simulink model "chirp_transmit"  (R2022a)
settings: Solver=FixedStepDiscrete  StartTime=0.0  StopTime=1  FixedStep=0.10000000000000001  RelTol=1e-3
model workspace (MAT data in the model file):
  imageBits = [0 1 0 1]
settings Model: Creator=luoch  LastModifiedBy=luoch
settings DataIOCC: SaveOutput=off  SignalLogging=off
settings ModelReferenceCC: EnableRefExpFcnMdlSchedulingChecks=off
settings RTWCC: Description=Generic Real-Time Target  GPUComputeCapability=5.0
settings ConfigComp: CovBoundaryAbsTol=1.0e-5

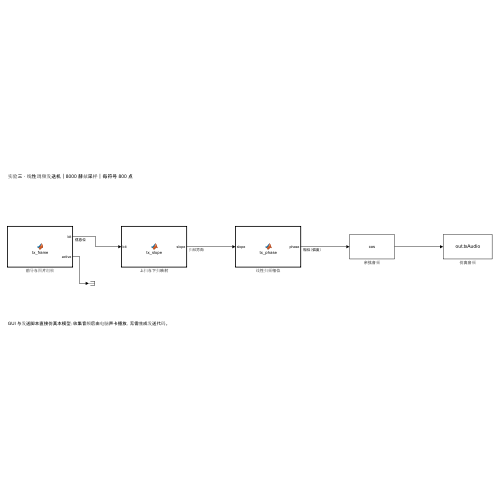
[thumbnail: Simulink's stored preview of the top-level diagram]
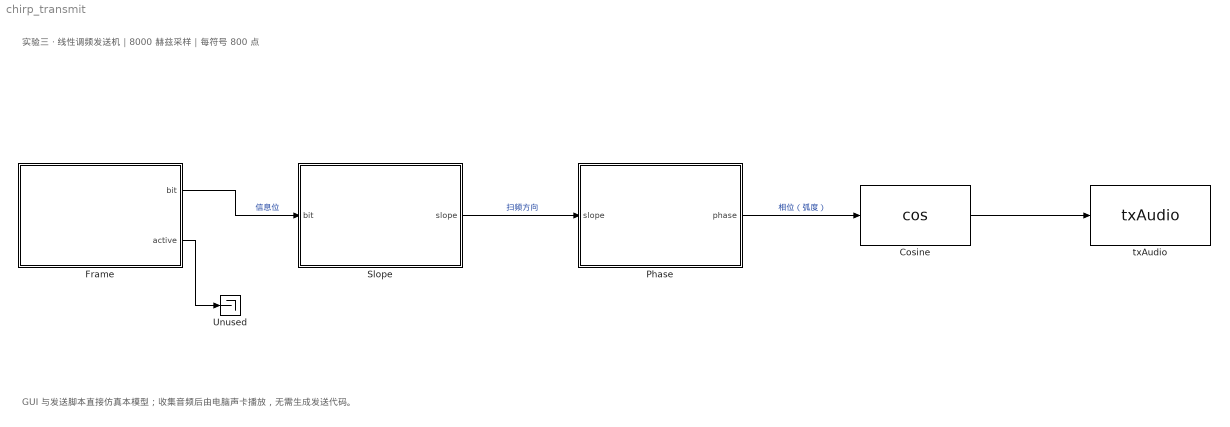
== system chirp_transmit ==
  note: 实验三 · 线性调频发送机｜8000 赫兹采样｜每符号 800 点
  note: GUI 与发送脚本直接仿真本模型；收集音频后由电脑声卡播放，无需生成发送代码。
  Cosine : Trigonometry  Operator=cos
      settings: AttributesFormatString=余弦音频
  Frame : MATLAB Function  TreatAsAtomicUnit=on
      settings: AttributesFormatString=前导与图片组帧
  Phase : MATLAB Function  TreatAsAtomicUnit=on
      settings: AttributesFormatString=线性扫频相位
  Slope : MATLAB Function  TreatAsAtomicUnit=on
      settings: AttributesFormatString=上扫与下扫映射
  Unused : Terminator
  txAudio : ToWorkspace  VariableName=txAudio  SampleTime=-1
      settings: AttributesFormatString=仿真音频
  wires:
  Frame/2(active) -> Unused/1
  Frame/1(bit) -> Slope/1(bit)  "信息位"
  Slope/1(slope) -> Phase/1(slope)  "扫频方向"
  Phase/1(phase) -> Cosine/1  "相位（弧度）"
  Cosine/1 -> txAudio/1

== matlab function chirp_transmit/Frame ==
  settings: updateMethod=DISCRETE  sampleTime=0.10000000000000001
  data: bit output; active output; imageBits parameter
function [bit,active]=tx_frame(imageBits)
%#codegen
% 前导、交替段、首尾 m 序列、图片比特及尾部保护，均在模型内产生。
persistent index
if isempty(index),index=1;end
mseq=[1 0 0 1 1 0 1 0 1 1 1 1 0 0 0];alternate=[1 0 1 0 1 0 1 0 1 0];
L=numel(imageBits);active=index<=50+L+5;bit=0;
if index>=11 && index<21,bit=alternate(index-10);
elseif index>=21 && index<36,bit=mseq(index-20);
elseif index>=36 && index<36+L,bit=imageBits(index-35);
elseif index>=36+L && index<51+L,bit=mseq(index-35-L);
end
index=index+1;
end

== matlab function chirp_transmit/Phase ==
  settings: updateMethod=DISCRETE  sampleTime=0.10000000000000001
  data: slope input; phase output
function phase=tx_phase(slope)
%#codegen
% 每符号从零相位开始；保留原实现的 800 点闭区间扫描网格。
t=linspace(0,.1,800)';phase=2*pi*1000*t+pi*slope*2000*t.^2;
end

== matlab function chirp_transmit/Slope ==
  settings: updateMethod=DISCRETE  sampleTime=0.10000000000000001
  data: bit input; slope output
function slope=tx_slope(bit)
%#codegen
% 比特零上扫，比特一下扫。
slope=1-2*bit;
end
